simulink model "AFTC_SIM"  (R2016a)
settings: Solver=VariableStepAuto  StartTime=0  StopTime=150  FixedStep=1  RelTol=1e-1
settings Model: Creator=mahmo  LastModifiedBy=mahmo

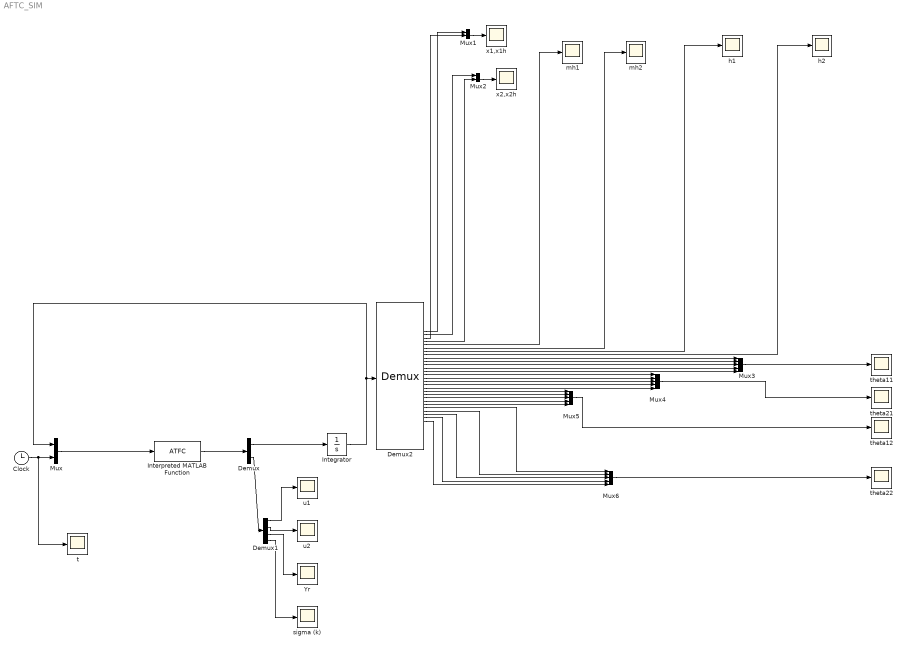
== system AFTC_SIM ==
  Clock : Clock
  Demux : Demux  Outputs="[28   4]"
  Demux1 : Demux  Outputs=[1 1 1 1]
  Demux2 : Demux  Outputs=[1 1 1 1 1 1 1 1 1 1 1 1 1 1 1 1 1 1 1 1 1 1 1 1 1 1 1 1]
  Integrator : Integrator  InitialCondition=[0.1 0.1 0 0 3.5 3.5 0 0 -0.1 -0.3 -0.5 -0.7 -0.9 0.1 0.3 0.5 0.7 0.9 -0.1 -0.3 -0.5 -0.7 -0.9 0.1 0.3 0.5 0.7 0.9]
  Interpreted MATLAB Function : MATLABFcn  MATLABFcn=ATFC  OutputDimensions=32
  Mux : Mux  Inputs=2
  Mux1 : Mux  Inputs=2
  Mux2 : Mux  Inputs=2
  Mux{3..6} (4 alike) : Mux  Inputs=5
  Yr : Scope
  h1 : Scope
  h2 : Scope
  mh1 : Scope
  mh2 : Scope
  sigma (k) : Scope
  t : Scope
  theta{11..12,21..22} (4 alike) : Scope
  u1 : Scope
  u2 : Scope
  "x1,x1h " : Scope
  x2,x2h : Scope
  wires:
  Interpreted MATLAB Function/1 -> Demux/1
  Clock/1 -> t/1, Mux/2
  Demux/2 -> Demux1/1
  Mux/1 -> Interpreted MATLAB Function/1
  Demux1/1 -> u1/1
  Demux1/2 -> u2/1
  Demux1/3 -> Yr/1
  Demux/1 -> Integrator/1
  Demux2/1 -> Mux1/1
  Demux2/3 -> Mux1/2
  Mux1/1 -> "x1,x1h "/1
  Mux2/1 -> x2,x2h/1
  Demux2/2 -> Mux2/1
  Demux2/4 -> Mux2/2
  Demux2/5 -> mh1/1
  Demux2/6 -> mh2/1
  Demux2/7 -> h1/1
  Demux2/8 -> h2/1
  Mux3/1 -> theta11/1
  Demux2/9 -> Mux3/1
  Demux2/10 -> Mux3/2
  Demux2/11 -> Mux3/3
  Demux2/12 -> Mux3/4
  Demux2/13 -> Mux3/5
  Demux2/14 -> Mux4/1
  Demux2/15 -> Mux4/2
  Demux2/16 -> Mux4/3
  Demux2/17 -> Mux4/4
  Demux2/18 -> Mux4/5
  Mux4/1 -> theta21/1
  Demux2/19 -> Mux5/1
  Demux2/20 -> Mux5/2
  Demux2/21 -> Mux5/3
  Demux2/22 -> Mux5/4
  Demux2/23 -> Mux5/5
  Demux2/24 -> Mux6/1
  Demux2/25 -> Mux6/2
  Demux2/26 -> Mux6/3
  Demux2/27 -> Mux6/4
  Demux2/28 -> Mux6/5
  Integrator/1 -> Demux2/1, Mux/1
  Mux5/1 -> theta12/1
  Mux6/1 -> theta22/1
  Demux1/4 -> sigma (k)/1
